simulink model "Outer_Tensor_Ex1"  (R2025a)
settings: Solver=VariableStepAuto  StartTime=0.0  StopTime=10  RelTol=1e-3
undefined symbols (not defined in the file): Correlation_ValidMode, DUT, L, vsva1596, xcvc1702
libraries: aieDSP x1, aieUtilities x1, vmcUtilities x1
settings Model: Creator=sdegala  LastModifiedBy=robg
settings ModelReferenceCC: EnableRefExpFcnMdlSchedulingChecks=on
settings RTWCC: GPUComputeCapability=3.5

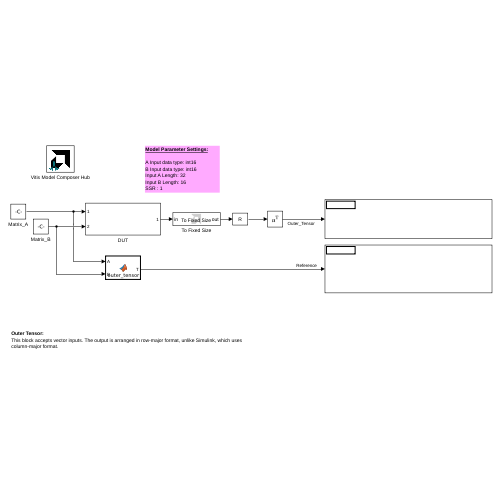
[thumbnail: Simulink's stored preview of the top-level diagram]
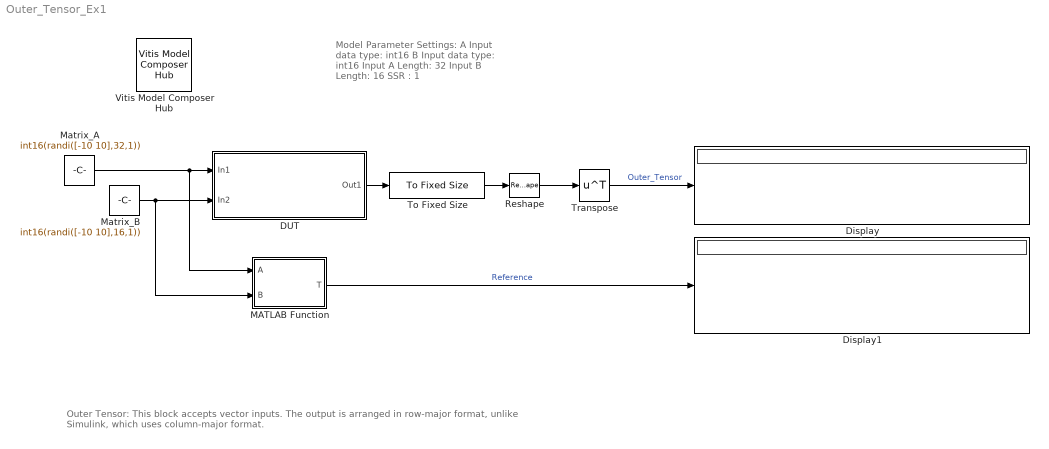
== system Outer_Tensor_Ex1 ==
  note: Outer Tensor:
      | This block accepts vector inputs. The output is arranged in row-major format, unlike Simulink, which uses column-major format.
  note: Model Parameter Settings:
      |
      | A Input data type: int16
      | B Input data type: int16
      | Input A Length: 32
      | Input B Length: 16
      | SSR : 1
  DUT : Subsystem
  Display : Display
  Display1 : Display
  MATLAB Function : MATLAB Function  TreatAsAtomicUnit=on
  Matrix_A : Constant  Value=int16(randi([-10 10],32,1))  OutDataTypeStr=int16  SampleTime=1
  Matrix_B : Constant  Value=int16(randi([-10 10],16,1))  OutDataTypeStr=int16  SampleTime=1
  Reshape : Reshape  OutputDimensionality=Customize  OutputDimensions=[16,32]
  To Fixed Size : aieUtilities/To Fixed Size  Mode=Stop simulation when input variable-size signal is not full  OutputSize=Inherit: Same as input  CopyMethod=Buffer samples to form output  HasStatusOutput=on
  Transpose : Math  Operator=transpose
  Vitis Model Composer Hub : vmcUtilities/Vitis Model Composer Hub  Tag=genX  CodeGeneration=off  SubsystemName=DUT  BlockHierPath=Correlation_ValidMode/DUT  SubsystemType=AIENode  StartColumn=1  NumberOfColumns=1  TargetDirectory=./code  exportDesign=off  analyzeDesign=on  validateDesignOnHw=off  ExportType=AI Engines  IpVendor=xilinx.com  IpLibrary=hls  IpVersion=1.0  IpHWLanguage=Verilog  AieCompilerOptions={}  AieSimulatorOptions={}  AieGraphIterations=-1  CreateTestbench=on  TestbenchStackSize=10  RunRtlSim=off  RunCSim=off  RunAieSim=off  AieSimTimeout=50000  RunAieSimProfiling=off  LaunchVitisAnalyzer=off  PlotOutput=off  RunX86Sim=off  X86SimTimeout=10  GenHwImage=off  GenLibadfXo=off  GenHwValidationCode=off  PlatformType=Not Specified  HwSystemType=Baremetal  HwValidationTarget=hw  ProjDevice=xcvc1702-vsva1596-2LP-e-L  ProjDevicePart=xcvc1702-vsva1596-2LP-e-L  AIEType=AIE  SamplePeriod=-1  ClockFrequency=200  DataPathParallelism=1  xilinxfamily=versalaicore  part=xcvc1702  speed=-2LP-e-L  package=vsva1596  directory=./netlist  testbench=off  incr_netlist=off  synthesis_tool=Vivado  clock_wrapper=Clock Enables  dbl_ovrd=According to Block Masks  dcm_input_clock_period=10  sysclk_period=10  simulink_period=1  eval_field=0  IPInfoJsonString="{\"DUTSubsystemName\":\"DUT\",\"AIESubsystem\":{\"SubsystemName\":\"DUT\",\"TargetDirectory\":\"./code\",\"AIEArrayConfig\":\"Use entire AIE array\",\"StartColumn\":\"0\",\"NumberOfColumns\":\"1\"},\"SubsystemTag\":\"AIENode\"}"  LogFileName=/proj/xhdhdstaff5/sdegala/Head1/HEAD/2025_2_work/AIE_BLOCKS_2025_2/code/model_composer.log  NThreads=4  IPConfigFile=/tmp/vmctmp-11198269997411262707/Correlation_ValidMode_ipconfig.json
  wires:
  DUT/1(Out1) -> To Fixed Size/1
  Matrix_A/1 -> DUT/1(In1), MATLAB Function/1(A)
  Matrix_B/1 -> DUT/2(In2), MATLAB Function/2(B)
  MATLAB Function/1(T) -> Display1/1  "Reference"
  Reshape/1 -> Transpose/1
  To Fixed Size/1 -> Reshape/1
  Transpose/1 -> Display/1  "Outer_Tensor"

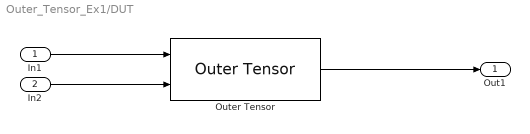
== system Outer_Tensor_Ex1/DUT ==
  In1 : Inport
  In2 : Inport  Port=2
  Outer Tensor : aieDSP/Outer Tensor  AIE_VARIANT=1  TP_API=0  data_type_A=int16  data_type_B=int16  dim_a=32  dim_b=16  num_frames=1  shift_output=0  ssr=1  rnd_mode=Floor  sat_mode=None  blockJsonConstraints=[]  blockJsonConstraintsInternal=[]  spec=vmc_outer_tensor.json  SerializedMaskParamNames=[]  SerializedMaskParamValues=[]  SerializedMaskParamVisibilities=[]  block_type=Outer Tensor  SerializedMaskParamDataypes=uint|uint|typename|typename|uint|uint|uint|uint|uint|uint|uint  SerializedMaskParamEnumStrArr=0|0|0|0|0|0|0|0|0|Floor,Ceiling,Round to positive infinity,Round to negative infinity,Round symmetrical to infinity,Round symmetrical to zero,Round convergent to even,Round convergent to odd|None,Saturate,Symmetric  SerializedMaskParamEnumValArr=0|0|0|0|0|0|0|0|0|0,1,2,3,4,5,6,7|0,1,3  SerializedMaskParamVectorArr=0|0|0|0|0|0|0|0|0|0|0  SerializedMaskParamKeys=AIE_VARIANT|TP_API|TT_DATA_A|TT_DATA_B|TP_DIM_A|TP_DIM_B|TP_NUM_FRAMES|TP_SHIFT|TP_SSR|TP_RND|TP_SAT
  Out1 : Outport
  wires:
  In2/1 -> Outer Tensor/2
  In1/1 -> Outer Tensor/1
  Outer Tensor/1 -> Out1/1

== matlab function Outer_Tensor_Ex1/MATLAB Function ==
  data: A input; T output; B input
function T = outer_tensor(A, B)
    szA = 32;
    szB = 16;

    Aexp = reshape(A, [szA ones(1,numel(szB))]);
    Bexp = reshape(B, [ones(1,numel(szA)) szB]);

    T = Aexp .* Bexp;
end
